simulink model "Copy_of_FaultFeeder"  (R2019a)
settings: Solver=ode1  StartTime=0.0  StopTime=2.5  FixedStep=Ts_Power  RelTol=1e-3
PostLoadFcn:
  | %% Init for wind PnO models - global system parameters
  | OVERRIDE_SSN_MEMORY_LIMIT=1;
  | Ts=50e-6;
  | % Ts=50e-10;
  | Ts_Power=Ts;
  | Ts_Control=2*Ts;
  | freq = 50;
  | Fnom=freq;
  | Vac=400e3;
InitFcn:
  | %% Init for wind PnO models - global system parameters
  | OVERRIDE_SSN_MEMORY_LIMIT=1;
  | Ts=50e-6;
  | % Ts=50e-10;
  | Ts_Power=Ts;
  | Ts_Control=2*Ts;
  | freq = 50;
  | Fnom=freq;
  | Vac=225e3;
values from neighbouring files (symbols this model uses):
  sub_posCap = sub_posCap*2.5    (= 4e-07)    [variable.m]
  sub_posInd = 0.001400563    [variable.m]
  sub_posR = 0.036    [variable.m]
  sub_zeroCap = sub_zeroCap*2.5    (= 1.333325e-07)    [variable.m]
  sub_zeroInd = 0.00420169    [variable.m]
  sub_zeroR = 0.108    [variable.m]
  transfo_L1 = 0.05999374    [variable.m]
  transfo_L2 = 0.05999374    [variable.m]
  transfo_R1 = 0.000866667    [variable.m]
  transfo_R2 = 0.00086667    [variable.m]
undefined symbols (not defined in the file or in its folder): D1, D11, Delta, den, DiscIntNeverNeededParam, dx, find_system, gcbh, num, out_Buses, out_WindFarms, sps_rtmsupport
libraries: powerlib x137, simulink x64, powerlib_meascontrol x64, elements x52, simulink_extras x38, eeSinusoidalMeasurement x35, spsVIMeasurementModel x27, eePowerMeasurement x11
(part 1 of 20)
settings Model: ARTEMISmethode_block_infos=$$__separator__$$  ExtModeAutoUpdateStatusClock=off  Creator=batserve  LastModifiedBy=sarah
settings SolverCC: AlgebraicLoopSolver=LineSearch  AutoInsertRateTranBlk=on
settings DataIOCC: SaveFormat=StructureWithTime  SaveOutput=off  InspectSignalLogs=on  SaveTime=off  ReturnWorkspaceOutputs=off
settings OptimizationCC: BlockReduction=off  ExpressionDepthLimit=2147483647  InitFltsAndDblsToZero=on  LifeSpan=inf
settings DebuggingCC: SaveWithParameterizedLinksMsg=none  UnderspecifiedInitializationDetection=Classic  MergeDetectMultiDrivingBlocksExec=none  SignalResolutionControl=TryResolveAllWithWarning  SolverPrmCheckMsg=warning  MultiTaskDSMMsg=warning  MultiTaskCondExecSysMsg=none  FcnCallInpInsideContextMsg=warning  StateNameClashWarn=warning  SFUnexpectedBacktrackingDiag=warning  SFNoUnconditionalDefaultTransitionDiag=warning  SFExecutionAtInitializationDiag=none  ArithmeticOperatorsInVariantConditions=warning
settings HardwareCC: ProdBitPerPointer=32  ProdBitPerSizeT=32  ProdBitPerPtrDiffT=32  ProdLargestAtomicFloat=None  ProdIntDivRoundTo=Undefined  ProdEndianess=Unspecified  ProdWordSize=32  ProdHWDeviceType=32-bit Generic  TargetHWDeviceType=32-bit Generic
settings ModelReferenceCC: PropagateSignalLabelsOutOfModel=off
settings SFSimCC: SimUseLocalCustomCode=off
settings RTWCC: RTWUseLocalCustomCode=off
settings CodeAppCC: StateflowObjectComments=on
settings GRTTargetCC: TargetFcnLib=ansi_tfl_tmw.mat  TargetLangStandard=C89/C90 (ANSI)  CombineOutputUpdateFcns=off  GRTInterface=on
settings ConfigComp: CovMetricSettings=dw  CovSaveCumulativeToWorkspaceVar=on  CovSaveSingleToWorkspaceVar=on  CovExternalEMLEnable=off  CovSFcnEnable=off
settings SimscapeCC: SimscapeNormalizeSystem=off

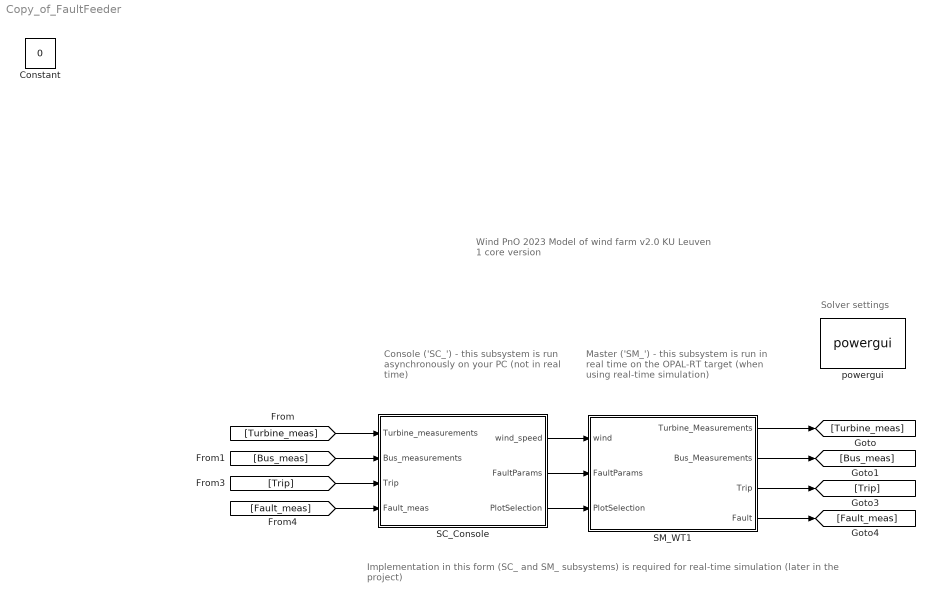
== system Copy_of_FaultFeeder ==
  note: Wind PnO 2023
      | Model of wind farm v2.0
      | KU Leuven
      | 1 core version
  note: Solver settings
  note: Master ('SM_') - this subsystem is run in real time on the OPAL-RT target (when using real-time simulation)
  note: Console ('SC_') - this subsystem is run asynchronously on your PC (not in real time)
  note: Implementation in this form (SC_ and SM_ subsystems) is required for real-time simulation (later in the project)
  SC_Console : Subsystem
  SM_WT1 : Subsystem
  powergui : powerlib/powergui  Priority=2  SimulationMode=Discrete  SampleTime=Ts  frequency=50  Iterations=50  frequencyindice=0  Pbase=100e6  ErrMax=1e-4  UnitsV=kV  UnitsW=MW  buscounter=0  FunctionMessages=off  echomessages=off  EnableUseOfTLC=off  CurrentSourceSwitches=off  DisableSnubberDevices=off  DisableRonSwitches=off  DisableVfSwitches=off  DisplayEquations=off  AutomaticDiscreteSolvers=off  SolverType=Backward Euler  Interpol=off  ExternalGateDelay=off  methode=off  Ts=0  x0status=blocks  SPID=off  SwTol=0  HookPort=off  NonlinearTolerance=1e-4  nMaxIteration=100  ContinueOnMaxIteration=off  RestoreLinks=warning  ResistiveCurrentMeasurement=off  Frange=[0:2:500]  Ylog=off  Xlog=on  ShowGrid=off  save=off  variable=ZData  structure=0  ZoomFFT=on  StartTime=0.0  cycles=1  DisplayStyle=1  fundamental=60  FreqAxis=off  MaxFrequency=1000  frequencyindicesteady=1  RmsSteady=1  display=off
      settings: SourceProductName=Simscape Electrical
  Constant : Constant  IOType=siggen  Value=0
  wires:
  SC_Console/1(wind_speed) -> SM_WT1/1(wind)
  SM_WT1/1(Turbine_Measurements) -> [Turbine_meas]
  SM_WT1/2(Bus_Measurements) -> [Bus_meas]
  [Turbine_meas] -> SC_Console/1(Turbine_measurements)
  [Bus_meas] -> SC_Console/2(Bus_measurements)
  SM_WT1/3(Trip) -> [Trip]
  [Trip] -> SC_Console/3(Trip)
  SM_WT1/4(Fault) -> [Fault_meas]
  [Fault_meas] -> SC_Console/4(Fault_meas)
  SC_Console/2("FaultParams ") -> SM_WT1/2("FaultParams ")
  SC_Console/3(PlotSelection) -> SM_WT1/3(PlotSelection)

== system Copy_of_FaultFeeder/SC_Console ==
  note: Inputs / Outputs
  note: Wind farm and bus visualization
  note: Wind farm and grid control
  note: CONTROL DASHBOARD
  note: WIND FARM
  note: BUS
  note: Wind Farm - Point of Connection
  note: Wind Farm - Wind turbine Converter (to be used for debugging purposes)
  note: Note that the wind turbine model does not represent the mechanical dynamics - only change the wind speed before the start of the simulation.
  note: FRT AND FAULT DISPLAYS
  note: FAULT MEASUREMENTS
  note: Select the bus and turbine for plotting here
  note: This subsystem is designed for monitoring. When performing real-time simulations, this is the only subsystem that you can view.
  Turbine_measurements : Inport
  Bus_measurements : Inport  Port=2
  Trip : Inport  Port=3
  Fault_meas : Inport  Port=4
  Bus Creator1 : BusCreator  Inputs=2
  Bus Creator2 : BusCreator  Inputs=2
  Bus Selector : BusSelector  OutputSignals=P (MW),Q (MVAr)  OutputAsBus=on
  Bus measurements : Scope  NumInputPorts=5
  Bus_Selection : Constant
  Disconnection display : Display
  FRT Disconnection Time (s) : Display
      settings: Format=bank
  Fault current abc and mag : Scope  NumInputPorts=2
  Grid Voltage and Grid code FRT requirements : Scope  NumInputPorts=2
  Grid-side Converter : Scope  NumInputPorts=4
  Minimum POC voltage (p.u.) : Display
      settings: Format=bank
  Peak POC current (p.u.) : Display
      settings: Format=bank
  Phase to ground measurements : Scope  NumInputPorts=4
  Rotor-side Converter : Scope  NumInputPorts=6
  Start time : Constant
  Subsystem : Subsystem
  Subsystem1 : Subsystem
  Subsystem3 : Subsystem
  Subsystem4 : Subsystem
  Tdrp : Constant  Value=10
  Time under FRT code requirements (s) : Display
      settings: Decimation=2
  Trip? : Display
      settings: Decimation=5000
  Visualization toolbox : Subsystem  Commented=on  mask(Visualization Toolbox){N_WindFarm=WindFarm_Selection_1, Visualization_save_windFarms=off, Visualization_save_windFarms_path='', GridSide_Scope=off, ConverterSide_Scope=off, DCSide_Scope=off, PhasetoGround_Scope=off, pu_Scope=off, FaultvsGridCode_Scope=off, Visualization_save_buses=off, Visualization_save_buses_path='', BusA_Scope=off, BusB_Scope=off, BusC_Scope=off, BusD_Scope=off, out_mask_WindFarms=out_WindFarms, out_mask_Buses=out_Buses}
      mask prompts: N_WindFarm "Select wind farm number"; Visualization_save_windFarms "Save figures?"; Visualization_save_windFarms_path "Enter file path for the figures"; GridSide_Scope "Grid Side"; ConverterSide_Scope "Converter Side"; DCSide_Scope "DC Side"; PhasetoGround_Scope "Phate to ground"; pu_Scope "p.u."; FaultvsGridCode_Scope "Fault vs. Grid code requirements"; Visualization_save_buses "Save figures?"; Visualization_save_buses_path "Enter file path for the figures"; BusA_Scope "Bus A"; BusB_Scope "Bus B"; BusC_Scope "Bus C"; BusD_Scope "Bus D"
      mask init:
      | %% Plot all graphs from the stored simulation output data according to the user's needs
      | 
      | % Import data
      | set_param(gcb,'out_mask_WindFarms','out_WindFarms');
      | set_param(gcb,'out_mask_Buses','out_Buses');
      | 
      | %% WindFarms
      | N_WindFarm=get_param(gcb,'N_WindFarm');
      | common_address=strcat('out_mask_WindFarms.',N_WindFarm,'.');
      | fontsize=20;
      | simul_stop_time=2;%%To be connected with get_param
      | close all
      | if GridSide_Scope
      |     figure
      |     end_address='WindTurbine_GridSide';
      |     address=strcat(common_address,end_address,'.');
      |     tiledlayout(4,1)
      |     %1
      |     final_address=strcat(address,'Vabc_grid__pu_');
      |     nexttile
      |     plot(eval(final_address));
      |     %Format
      |     xlabel('Time (s)','FontSize', fontsize-8);
      |     ylabel('V_a_b_c grid (p.u.)','FontSize', fontsize-8);
      |     title(strcat(N_WindFarm,' - V_a_b_c grid (p.u.)'),'FontSize', fontsize-5);
      |     xlim([0 simul_stop_time])
      |     %2
      |     final_address=strcat(address,'Iabc_conv__pu_');
      |     nexttile
      |     plot(eval(final_address));
      |     %Format
      |     xlabel('Time (s)','FontSize', fontsize-8);
      |     ylabel('I_a_b_c grid (p.u.)','FontSize', fontsize-8);
      |     title(strcat(N_WindFarm,' - I_a_b_c grid (p.u.)'),'FontSize', fontsize-5);
      |     xlim([0 simul_stop_time])
      |     %3
      |     final_address=strcat(address,'P_grid');
      |     nexttile
      |     plot(eval(final_address));
      |     %Format
      |     xlabel('Time (s)','FontSize', fontsize-8);
      |     ylabel('P grid (p.u.)','FontSize', fontsize-8);
      |     title(strcat(N_WindFarm,' - P grid (p.u.)'),'FontSize', fontsize-5);
      |     xlim([0 simul_stop_time])
      |     %4
      |     final_address=strcat(address,'Q_grid');
      |     nexttile
      |     plot(eval(final_address));
      |     %Format
      |     xlabel('Time (s)','FontSize', fontsize-8);
      |     ylabel('Q grid (p.u.)','FontSize', fontsize-8);
      |     title(strcat(N_WindFarm,' - Q grid (p.u.)'),'FontSize', fontsize-5);
      |     xlim([0 simul_stop_time])
      |  
      |     %Save figure
      |     if Visualization_save_windFarms
      |         file_name=strcat(N_WindFarm,'_','Grid_side_scope');
      |         saveas(gca, fullfile(Visualization_save_windFarms_path, file_name), 'fig');
      |     end
      | end
      | 
      | if ConverterSide_Scope
      |     figure
      |     end_address='WindTurbine_ConverterSide';
      |     address=strcat(common_address,end_address,'.');
      |     tiledlayout(6,1)
      |     %1
      |     final_address=strcat(address,'Q_grid__y__nom__b__measured_');
      |     nexttile
      |     plot(eval(final_address));
      |     %Format
      |     xlabel('Time (s)','FontSize', fontsize-8);
      |     ylabel('Q grid nom and measured','FontSize', fontsize-8);%%%%%%%%%%%%%
      |     title(strcat(N_WindFarm,' - Q grid nom and measured'),'FontSize', fontsize-5);
      |     xlim([0 simul_stop_time])
      |     %2
      |     final_address=strcat(address,'V_dc__y__nom__b__measured_');
      |     nexttile
      |     plot(eval(final_address));
      |     %Format
      |     xlabel('Time (s)','FontSize', fontsize-8);
      |     ylabel('V_D_C nom and measured','FontSize', fontsize-8);
      |     title(strcat(N_WindFarm,' - V_D_C nom and measured'),'FontSize', fontsize-5);%%%%%%%%%%%%%
      |     xlim([0 simul_stop_time])
      |     %3
      |     final_address=strcat(address,'I_abc__A_');
      |     nexttile
      |     plot(eval(final_address));
      |     %Format
      |     xlabel('Time (s)','FontSize', fontsize-8);
      |     ylabel('I_a_b_c (A)','FontSize', fontsize-8);
      |     title(strcat(N_WindFarm,' - I_a_b_c'),'FontSize', fontsize-5);
      |     xlim([0 simul_stop_time])
      |     %4
      |     final_address=strcat(address,'id');
      |     nexttile
      |     plot(eval(final_address));
      |     %Format
      |     xlabel('Time (s)','FontSize', fontsize-8);
      |     ylabel('id','FontSize', fontsize-8);
      |     title(strcat(N_WindFarm,' - id'),'FontSize', fontsize-5);
      |     xlim([0 simul_stop_time])
      |     %5
      |     final_address=strcat(address,'iq');
      |     nexttile
      |     plot(eval(final_address));
      |     %Format
      |     xlabel('Time (s)','FontSize', fontsize-8);
      |     ylabel('iq','FontSize', fontsize-8);
      |     title(strcat(N_WindFarm,' - iq'),'FontSize', fontsize-5);
      |     xlim([0 simul_stop_time])
      |     %6
      |     final_address=strcat(address,'theta_PLL');%%%%%%%%%%%%
      |     nexttile
      |     plot(eval(final_address));
      |     %Format
      |     xlabel('Time (s)','FontSize', fontsize-8);
      |     ylabel('theta_P_L_L','FontSize', fontsize-8);
      |     title(strcat(N_WindFarm,' - theta_P_L_L'),'FontSize', fontsize-5);
      |     xlim([0 simul_stop_time])
      |     %Save figure
      |     if Visualization_save_windFarms
      |         file_name=strcat(N_WindFarm,'_','Converter_side_scope');
      |         saveas(gca, fullfile(Visualization_save_windFarms_path, file_name), 'fig');
      |     end
      | end
      | 
      | if DCSide_Scope
      |     figure
      |     end_address='WindTurbine_DCSide';
      |     address=strcat(common_address,end_address,'.');
      |     tiledlayout(4,1)
      |     %1
      |     nexttile
      |     hold on
      |     final_address=strcat(address,'Idc_gen_grid.Idc_gen');
      |     plot(eval(final_address));
      |     final_address=strcat(address,'Idc_gen_grid.Idc_grid');
      |     plot(eval(final_address));
      |     %Format
      |     xlabel('Time (s)','FontSize', fontsize-8);
      |     ylabel('I_DC gen and I_DC grid','FontSize', fontsize-8);
      |     title(strcat(N_WindFarm,' - I_DC gen and I_DC grid'),'FontSize', fontsize-5);
      |     xlim([0 simul_stop_time])
      |     hold off
      |     %2
      |     nexttile
      |     hold on
      |     final_address=strcat(address,'I_cap_chopper.I_cap');
      |     plot(eval(final_address));
      |     final_address=strcat(address,'I_cap_chopper.I_chopper');
      |     plot(eval(final_address));
      |     %Format
      |     xlabel('Time (s)','FontSize', fontsize-8);
      |     ylabel('Icap and Ichopper','FontSize', fontsize-8);
      |     title(strcat(N_WindFarm,' - Icap and Ichopper'),'FontSize', fontsize-5);
      |     xlim([0 simul_stop_time])
      |     hold off
      |     %3
      |     final_address=strcat(address,'Pgrid');
      |     nexttile
      |     plot(eval(final_address));
      |     %Format
      |     xlabel('Time (s)','FontSize', fontsize-8);
      |     ylabel('P_g_r_i_d','FontSize', fontsize-8);
      |     title(strcat(N_WindFarm,' - P_g_r_i_d'),'FontSize', fontsize-5);
      |     xlim([0 simul_stop_time])
      |     %4
      |     final_address=strcat(address,'vdc');
      |     nexttile
      |     plot(eval(final_address));
      |     %Format
      |     xlabel('Time (s)','FontSize', fontsize-8);
      |     ylabel('V_D_C','FontSize', fontsize-8);
      |     title(strcat(N_WindFarm,' - V_D_C'),'FontSize', fontsize-5);
      |     xlim([0 simul_stop_time])
      |     %Save figure
      |     if Visualization_save_windFarms
      |         file_name=strcat(N_WindFarm,'_','DC_side_scope');
      |         saveas(gca, fullfile(Visualization_save_windFarms_path, file_name), 'fig');
      |     end
      | end
      | 
      | if PhasetoGround_Scope
      |     figure
      |     end_address='WindTurbine_PhasetoGroundMeasurements';
      |     address=strcat(common_address,end_address,'.');
      |     tiledlayout(3,1)
      |     %1
      |     nexttile
      |     final_address=strcat(address,'Vabc__kV_');
      |     plot(eval(final_address));
      |     %Format
      |     xlabel('Time (s)','FontSize', fontsize-8);
      |     ylabel('V_a_b_c (kV)','FontSize', fontsize-8);
      |     title(strcat(N_WindFarm,' - V_a_b_c (kV)'),'FontSize', fontsize-5);
      |     xlim([0 simul_stop_time])
      |     %2
      |     nexttile
      |     final_address=strcat(address,'Iabc');
      |     plot(eval(final_address));
      |     %Format
      |     xlabel('Time (s)','FontSize', fontsize-8);
      |     ylabel('I_a_b_c (A)','FontSize', fontsize-8);
      |     title(strcat(N_WindFarm,' - I_a_b_c (A)'),'FontSize', fontsize-5);
      |     xlim([0 simul_stop_time])
      |     %3
      |     nexttile
      |     hold on
      |     final_address=strcat(address,'PQ.P__MW_');
      |     plot(eval(final_address));
      |     final_address=strcat(address,'PQ.Q__MVA_');
      |     plot(eval(final_address));
      |     final_address=strcat(address,'Pelec__MW_');
      |     plot(eval(final_address));
      |     %Format
      |     xlabel('Time (s)','FontSize', fontsize-8);
      |     ylabel('P (MW) and Q (MVAr)','FontSize', fontsize-8);
      |     title(strcat(N_WindFarm,' - P (MW) and Q (MVAr)'),'FontSize', fontsize-5);
      |     xlim([0 simul_stop_time])
      |     hold off
      |     %Save figure
      |     if Visualization_save_windFarms
      |         file_name=strcat(N_WindFarm,'_','Phase_to_ground_scope');
      |         saveas(gca, fullfile(Visualization_save_windFarms_path, file_name), 'fig');
      |     end
      | end
      | 
      | if pu_Scope
      |     figure
      |     end_address='WindTurbine_puMeasurements';
      |     address=strcat(common_address,end_address,'.');
      |     tiledlayout(3,1)
      |     %1
      |     nexttile
      |     final_address=strcat(address,'Vabc_pu_mag');
      |     plot(eval(final_address));
      |     %Format
      |     xlabel('Time (s)','FontSize', fontsize-8);
      |     ylabel('V_a_b_c mag (p.u.)','FontSize', fontsize-8);
      |     title(strcat(N_WindFarm,' - V_a_b_c mag (p.u.)'),'FontSize', fontsize-5);
      |     xlim([0 simul_stop_time])
      |     %2
      |     nexttile
      |     final_address=strcat(address,'Iabc_pu_mag');
      |     plot(eval(final_address));
      |     %Format
      |     xlabel('Time (s)','FontSize', fontsize-8);
      |     ylabel('I_a_b_c mag (p.u.)','FontSize', fontsize-8);
      |     title(strcat(N_WindFarm,' - I_a_b_c mag (p.u.)'),'FontSize', fontsize-5);
      |     xlim([0 simul_stop_time])
      |     %3
      |     nexttile
      |     hold on
      |     final_address=strcat(address,'PQ.P_pu');
      |     plot(eval(final_address));
      |     final_address=strcat(address,'PQ.Q_pu');
      |     plot(eval(final_address));
      |     final_address=strcat(address,'Pelec_pu');
      |     plot(eval(final_address));
      |     %Format
      |     xlabel('Time (s)','FontSize', fontsize-8);
      |     ylabel('P (p.u.) and Q (p.u.)','FontSize', fontsize-8);
      |     title(strcat(N_WindFarm,' - P (p.u.) and Q (p.u.)'),'FontSize', fontsize-5);
      |     xlim([0 simul_stop_time])
      |     hold off
      |     %Save figure
      |     if Visualization_save_windFarms
      |         file_name=strcat(N_WindFarm,'_','pu_scope');
      |         saveas(gca, fullfile(Visualization_save_windFarms_path, file_name), 'fig');
      |     end
      | end
      | 
      | if FaultvsGridCode_Scope
      |     figure
      |     end_address='Windturbine_FaultvsGridFRTRequirements';
      |     address=strcat(common_address,end_address,'.');
      |     %1
      |     hold on
      |     final_address=strcat(address,'Vabc_pu_mag');
      |     plot(eval(final_address));
      |     final_address=strcat(address,'Grid_Code_FRT_requirements');
      |     plot(eval(final_address));
      |     xlabel('Time (s)','FontSize', fontsize-8);
      |     ylabel('V (p.u.) - Fault vs Grid FRT Requirements','FontSize', fontsize-8);
      |     title(strcat(N_WindFarm,' - V (p.u.) - Fault vs Grid FRT Requirements'),'FontSize', fontsize-5);
      |     xlim([0 simul_stop_time])
      |     hold off
      |     %Save figure
      |     if Visualization_save_windFarms
      |         file_name=strcat(N_WindFarm,'_','Fault_vs_Grid_code_scope');
      |         saveas(gca, fullfile(Visualization_save_windFarms_path, file_name), 'fig');
      |     end
      | end
      | 
      | %% Buses
      | 
      | common_address=strcat('out_mask_Buses.');
      | 
      | if BusA_Scope
      |     figure
      |     end_address='BusA';
      |     address=strcat(common_address,end_address,'.');
      |     tiledlayout(5,1)
      |     %1
      |     nexttile
      |     final_address=strcat(address,'Vabc');
      |     plot(eval(final_address));
      |     %Format
      |     xlabel('Time (s)','FontSize', fontsize-8);
      |     ylabel('Vabc (kV)','FontSize', fontsize-8);
      |     title(strcat(end_address,' - Vabc', fontsize-5));
      |     xlim([0 simul_stop_time])
      |     %2
      |     nexttile
      |     final_address=strcat(address,'Iabc');
      |     plot(eval(final_address));
      |     %Format
      |     xlabel('Time (s)','FontSize', fontsize-8);
      |     ylabel('Iabc (A)','FontSize', fontsize-8);
      |     title(strcat(end_address,' - Iabc', fontsize-5));
      |     xlim([0 simul_stop_time])
      |     %3
      |     nexttile
      |     final_address=strcat(address,'V_mag');
      |     plot(eval(final_address));
      |     %Format
      |     xlabel('Time (s)','FontSize', fontsize-8);
      |     ylabel('V_m_a_g (kV)','FontSize', fontsize-8);
      |     title(strcat(end_address,' - V_m_a_g','FontSize',fontsize-5));
      |     xlim([0 simul_stop_time])
      |     %4
      |     final_address=strcat(address,'I_mag');
      |     nexttile
      |     plot(eval(final_address));
      |     %Format
      |     xlabel('Time (s)','FontSize', fontsize-8);
      |     ylabel('I_m_a_g (A)','FontSize', fontsize-8);
      |     title(strcat(end_address,' - I_m_a_g','FontSize',fontsize-5));
      |     xlim([0 simul_stop_time])
      |     %5
      |     nexttile
      |     hold on
      |     final_address=strcat(address,'PQ.P__MW_');
      |     plot(eval(final_address));
      |     final_address=strcat(address,'PQ.Q__MVAr_');
      |     plot(eval(final_address));
      |     %Format
      |     xlabel('Time (s)','FontSize', fontsize-8);
      |     ylabel('P (MW) and Q (MVAr)','FontSize', fontsize-8);
      |     title(strcat(end_address,' - P and Q','FontSize',fontsize-5));
      |     xlim([0 simul_stop_time])
      |     hold off
      | 
      |     %Save figure
      |     if Visualization_save_buses
      |         file_name='BusA_scope';
      |         saveas(gca, fullfile(Visualization_save_buses_path, file_name), 'fig');
      |     end
      | end
      | 
      | if BusB_Scope
      |     figure
      |     end_address='BusB';
      |     address=strcat(common_address,end_address,'.');
      |     tiledlayout(5,1)
      |     %1
      |     nexttile
      |     final_address=strcat(address,'Vabc');
      |     plot(eval(final_address));
      |     %Format
      |     xlabel('Time (s)','FontSize', fontsize-8);
      |     ylabel('Vabc (kV)','FontSize', fontsize-8);
      |     title(strcat(end_address,' - Vabc', fontsize-5));
      |     xlim([0 simul_stop_time])
      |     %2
      |     nexttile
      |     final_address=strcat(address,'Iabc');
      |     plot(eval(final_address));
      |     %Format
      |     xlabel('Time (s)','FontSize', fontsize-8);
      |     ylabel('Iabc (A)','FontSize', fontsize-8);
      |     title(strcat(end_address,' - Iabc', fontsize-5));
      |     xlim([0 simul_stop_time])
      |     %3
      |     nexttile
      |     final_address=strcat(address,'V_mag');
      |     plot(eval(final_address));
      |     %Format
      |     xlabel('Time (s)','FontSize', fontsize-8);
      |     ylabel('V_m_a_g (kV)','FontSize', fontsize-8);
      |     title(strcat(end_address,' - V_m_a_g','FontSize',fontsize-5));
      |     xlim([0 simul_stop_time])
      |     %4
      |     final_address=strcat(address,'I_mag');
      |     nexttile
      |     plot(eval(final_address));
      |     %Format
      |     xlabel('Time (s)','FontSize', fontsize-8);
      |     ylabel('I_m_a_g (A)','FontSize', fontsize-8);
      |     title(strcat(end_address,' - I_m_a_g','FontSize',fontsize-5));
      |     xlim([0 simul_stop_time])
      |     %5
      |     nexttile
      |     hold on
      |     final_address=strcat(address,'PQ.P__MW_');
      |     plot(eval(final_address));
      |     final_address=strcat(address,'PQ.Q__MVAr_');
      |     plot(eval(final_address));
      |     %Format
      |     xlabel('Time (s)','FontSize', fontsize-8);
      |     ylabel('P (MW) and Q (MVAr)','FontSize', fontsize-8);
      |     title(strcat(end_address,' - P and Q','FontSize',fontsize-5));
      |     xlim([0 simul_stop_time])
      |     hold off
      | 
      |     %Save figure
      |     if Visualization_save_buses
      |         file_name='BusB_scope';
      |         saveas(gca, fullfile(Visualization_save_buses_path, file_name), 'fig');
      |     end
      | end
      | 
      | if BusC_Scope
      |     figure
      |     end_address='BusC';
      |     address=strcat(common_address,end_address,'.');
      |     tiledlayout(5,1)
      |     %1
      |     nexttile
      |     final_address=strcat(address,'Vabc');
      |     plot(eval(final_address));
      |     %Format
      |     xlabel('Time (s)','FontSize', fontsize-8);
      |     ylabel('Vabc (kV)','FontSize', fontsize-8);
      |     title(strcat(end_address,' - Vabc', fontsize-5));
      |     xlim([0 simul_stop_time])
      |     %2
      |     nexttile
      |     final_address=strcat(address,'Iabc');
      |     plot(eval(final_address));
      |     %Format
      |     xlabel('Time (s)','FontSize', fontsize-8);
      |     ylabel('Iabc (A)','FontSize', fontsize-8);
      |     title(strcat(end_address,' - Iabc', fontsize-5));
      |     xlim([0 simul_stop_time])
      |     %3
      |     nexttile
      |     final_address=strcat(address,'V_mag');
      |     plot(eval(final_address));
      |     %Format
      |     xlabel('Time (s)','FontSize', fontsize-8);
      |     ylabel('V_m_a_g (kV)','FontSize', fontsize-8);
      |     title(strcat(end_address,' - V_m_a_g','FontSize',fontsize-5));
      |     xlim([0 simul_stop_time])
      |     %4
      |     final_address=strcat(address,'I_mag');
      |     nexttile
      |     plot(eval(final_address));
      |     %Format
      |     xlabel('Time (s)','FontSize', fontsize-8);
      |     ylabel('I_m_a_g (A)','FontSize', fontsize-8);
      |     title(strcat(end_address,' - I_m_a_g','FontSize',fontsize-5));
      |     xlim([0 simul_stop_time])
      |     %5
      |     nexttile
      |     hold on
      |     final_address=strcat(address,'PQ.P__MW_');
      |     plot(eval(final_address));
      |     final_address=strcat(address,'PQ.Q__MVAr_');
      |     plot(eval(final_address));
      |     %Format
      |     xlabel('Time (s)','FontSize', fontsize-8);
      |     ylabel('P (MW) and Q (MVAr)','FontSize', fontsize-8);
      |     title(strcat(end_address,' - P and Q','FontSize',fontsize-5));
      |     xlim([0 simul_stop_time])
      |     hold off
      | 
      |     %Save figure
      |     if Visualization_save_buses
      |         file_name='BusC_scope';
      |         saveas(gca, fullfile(Visualization_save_buses_path, file_name), 'fig');
      |     end
      | end
      | 
      | if BusD_Scope
      |     figure
      |     end_address='BusD';
      |     address=strcat(common_address,end_address,'.');
      |     tiledlayout(5,1)
      |     %1
      |     nexttile
      |     final_address=strcat(address,'Vabc');
      |     plot(eval(final_address));
      |     %Format
      |     xlabel('Time (s)','FontSize', fontsize-8);
      |     ylabel('Vabc (kV)','FontSize', fontsize-8);
      |     title(strcat(end_address,' - Vabc', fontsize-5));
      |     xlim([0 simul_stop_time])
      |     %2
      |     nexttile
      |     final_address=strcat(address,'Iabc');
      |     plot(eval(final_address));
      |     %Format
      |     xlabel('Time (s)','FontSize', fontsize-8);
      |     ylabel('Iabc (A)','FontSize', fontsize-8);
      |     title(strcat(end_address,' - Iabc', fontsize-5));
      |     xlim([0 simul_stop_time])
      |     %3
      |     nexttile
      |     final_address=strcat(address,'V_mag');
      |     plot(eval(final_address));
      |     %Format
      |     xlabel('Time (s)','FontSize', fontsize-8);
      |     ylabel('V_m_a_g (kV)','FontSize', fontsize-8);
      |     title(strcat(end_address,' - V_m_a_g','FontSize',fontsize-5));
      |     xlim([0 simul_stop_time])
      |     %4
      |     final_address=strcat(address,'I_mag');
      |     nexttile
      |     plot(eval(final_address));
      |     %Format
      |     xlabel('Time (s)','FontSize', fontsize-8);
      |     ylabel('I_m_a_g (A)','FontSize', fontsize-8);
      |     title(strcat(end_address,' - I_m_a_g','FontSize',fontsize-5));
      |     xlim([0 simul_stop_time])
      |     %5
      |     nexttile
      |     hold on
      |     final_address=strcat(address,'PQ.P__MW_');
      |     plot(eval(final_address));
      |     final_address=strcat(address,'PQ.Q__MVAr_');
      |     plot(eval(final_address));
      |     %Format
      |     xlabel('Time (s)','FontSize', fontsize-8);
      |     ylabel('P (MW) and Q (MVAr)','FontSize', fontsize-8);
      |     title(strcat(end_address,' - P and Q','FontSize',fontsize-5));
      |     xlim([0 simul_stop_time])
      |     hold off
      | 
      |     %Save figure
      |     if Visualization_save_buses
      |         file_name='BusD_scope';
      |         saveas(gca, fullfile(Visualization_save_buses_path, file_name), 'fig');
      |     end
      | end
      mask Help:
      | Enter folder path between ' '.
      | e.g.
      | 'C:\Users\X\Desktop\Parent path\Case 1'
      mask TypeOptions N_WindFarm: WindFarm_Selection_1 | WindFarm_Selection_2 | WindFarm_Selection_3 | WindFarm_Selection_4 | WindFarm_Selection_5 | WindFarm_Selection_6 | WindFarm_Selection_7 | WindFarm_Selection_8 | WindFarm_Selection_9 | WindFarm_Selection_10
      mask DialogControl DescGroupVar Prompt: Visualization Toolbox
      mask DialogControl DescTextVar Prompt: This mask is used to select which data packs are printed on the scopes and saved as figures
      mask DialogControl Container5 Prompt: WindFarms
      mask DialogControl Scope_Selector Prompt: Select the variable pack to print
      mask DialogControl Container10 Prompt: Buses
      mask DialogControl Container11 Prompt: Select buses to print
      mask Display: image('VisualizationToolbox1.png')
  Wind speed (m/s) : Constant  Value=23
  WindTurbine_Selection : Constant
  pu measurements : Scope  NumInputPorts=4
  wind_speed : Outport  VectorParamsAs1DForOutWhenUnconnected=on
  "FaultParams " : Outport  Port=2  VectorParamsAs1DForOutWhenUnconnected=on
  PlotSelection : Outport  Port=3  VectorParamsAs1DForOutWhenUnconnected=on
  wires:
  Wind speed (m/s)/1 -> wind_speed/1
  [trip] -> Trip?/1
  [Iabc] -> Phase to ground measurements/2
  [Pelec] -> Phase to ground measurements/4
  [PQ] -> Phase to ground measurements/3
  [Vabc_kV] -> Phase to ground measurements/1
  [Vabc_pu_mag] -> pu measurements/1
  [Iabc_pu_mag] -> pu measurements/2
  [PQ_pu] -> pu measurements/3
  [Pelec_pu] -> pu measurements/4
  [Minimum_Voltage_pu] -> Minimum POC voltage (p.u.)/1  "Minimum Voltage pu"
  [FRT_disconnection_time] -> FRT Disconnection Time (s)/1  "FRT Disconnection Time"
  [Peak_POC_current_pu] -> Peak POC current (p.u.)/1  "Peak POC Current pu"
  [FRT_time] -> Time under FRT code requirements (s)/1  "Time under FRT"
  [Disconnection_trigger] -> Subsystem3/1(Disconnection_Trigger)
  Subsystem3/1(Disconnection message) -> Disconnection display/1
  [Vabc_grid_pu] -> Grid-side Converter/1
  [Iabc_conv_pu] -> Grid-side Converter/2
  [Pgrid] -> Grid-side Converter/3
  [Qgrid] -> Grid-side Converter/4
  [Qgrid_nomandmeas] -> Rotor-side Converter/1
  [Vdc_nomandmeas] -> Rotor-side Converter/2
  [Iabc_ref] -> Rotor-side Converter/3
  [Theta_PLL] -> Rotor-side Converter/6
  [Bus_Vabc] -> Bus measurements/1
  [Bus_PQ] -> Bus Selector/1
  [Bus_Imag] -> Bus measurements/4
  [Bus_Vmag] -> Bus measurements/3
  [Bus_Iabc] -> Bus measurements/2
  [Vabc_pu_mag] -> Grid Voltage and Grid code FRT requirements/1
  [FRT_grid_code_requirements] -> Grid Voltage and Grid code FRT requirements/2
  [id] -> Rotor-side Converter/4
  [iq] -> Rotor-side Converter/5
  [Fault_meas] -> Subsystem4/1(Fault Current abc)  "Fault Current abc"
  Subsystem4/1(Fault Current mag (kA)) -> Fault current abc and mag/1
  Subsystem4/2(Fault Current abc (kA)) -> Fault current abc and mag/2
  Turbine_measurements/1 -> Subsystem/1(In1)
  Bus_measurements/1 -> Subsystem1/1(In1)
  Trip/1 -> [trip]
  Fault_meas/1 -> [Fault_meas]
  Bus Creator1/1 -> "FaultParams "/1
  Start time/1 -> Bus Creator1/1  "start_time"
  Tdrp/1 -> Bus Creator1/2  "duration"
  Bus Selector/1 -> Bus measurements/5
  Bus Creator2/1 -> PlotSelection/1
  WindTurbine_Selection/1 -> Bus Creator2/1  "Turbine"
  Bus_Selection/1 -> Bus Creator2/2  "Bus"
